simulink model "LFCSsimulink"  (R2015b)
settings: Solver=VariableStepAuto  StartTime=0.0  StopTime=40  RelTol=1e-3
libraries: simulink x1
settings Model: PauseTimes=1  Creator=Vamshi  LastModifiedBy=Vamshi

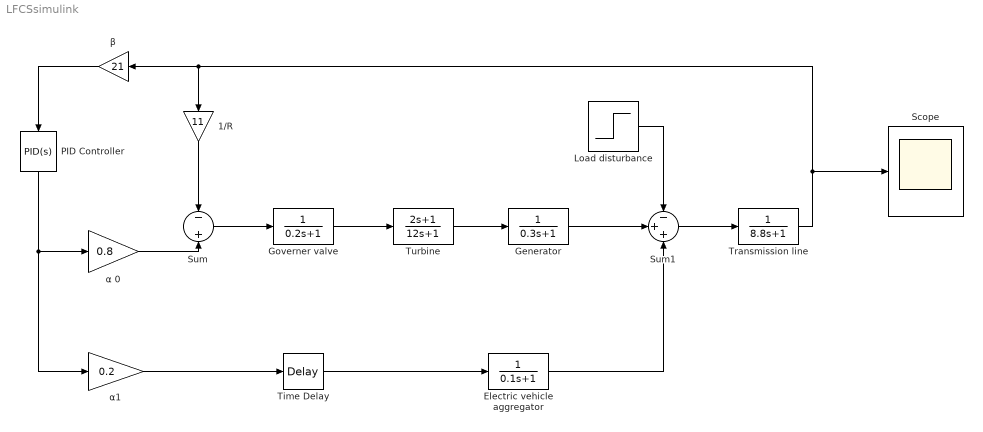
== system LFCSsimulink ==
  1/R : Gain  Gain=11
  Electric vehicle aggregator : TransferFcn  Denominator=[0.1 1]
  Generator : TransferFcn  Denominator=[0.3 1]
  Governer valve : TransferFcn  Denominator=[0.2 1]
  Load disturbance : Step  Time=0  After=.04  SampleTime=0
  PID Controller : simulink/Continuous/PID Controller  Controller=PID  TimeDomain=Continuous-time  SampleTime=-1  IntegratorMethod=Forward Euler  FilterMethod=Forward Euler  Form=Parallel  UseFilter=on  ControllerParametersSource=internal  P=-4  I=-2  D=0  N=100  InitialConditionSource=internal  InitialConditionForIntegrator=0  InitialConditionForFilter=0  ExternalReset=none  LimitOutput=off  UpperSaturationLimit=inf  LowerSaturationLimit=-inf  LinearizeAsGain=on  AntiWindupMode=none  Kb=1  TrackingMode=off  Kt=1  PParamMin=[]  PParamMax=[]  IParamMin=[]  IParamMax=[]  DParamMin=[]  DParamMax=[]  NParamMin=[]  NParamMax=[]  KbParamMin=[]  KbParamMax=[]  KtParamMin=[]  KtParamMax=[]  POutMin=[]  POutMax=[]  IOutMin=[]  IOutMax=[]  DOutMin=[]  DOutMax=[]  NOutMin=[]  NOutMax=[]  KbOutMin=[]  KbOutMax=[]  KtOutMin=[]  KtOutMax=[]  IntegratorOutMin=[]  IntegratorOutMax=[]  FilterOutMin=[]  FilterOutMax=[]  SumOutMin=[]  SumOutMax=[]  SumI1OutMin=[]  SumI1OutMax=[]  SumI2OutMin=[]  SumI2OutMax=[]  SumI3OutMin=[]  SumI3OutMax=[]  SumDOutMin=[]  SumDOutMax=[]  SaturationOutMin=[]  SaturationOutMax=[]  IntegratorContinuousStateAttributes=''  IntegratorStateMustResolveToSignalObject=off  IntegratorRTWStateStorageClass=Auto  FilterContinuousStateAttributes=''  FilterStateMustResolveToSignalObject=off  FilterRTWStateStorageClass=Auto  DifferentiatorICPrevScaledInput=0  DifferentiatorOutMin=[]  DifferentiatorOutMax=[]
  Scope : Scope
  Sum : Sum  Inputs=-+
  Sum1 : Sum  Inputs=-++
  Time Delay : TransportDelay  DelayTime=0.5  PadeOrder=5
  Transmission line : TransferFcn  Denominator=[8.8 1]
  Turbine : TransferFcn  Numerator=[2 1]  Denominator=[12 1]
  α 0 : Gain  Gain=0.8
  α1 : Gain  Gain=0.2
  β : Gain  Gain=21
  wires:
  Sum/1 -> Governer valve/1
  Governer valve/1 -> Turbine/1
  Turbine/1 -> Generator/1
  Generator/1 -> Sum1/2
  Sum1/1 -> Transmission line/1
  Load disturbance/1 -> Sum1/1
  α1/1 -> Time Delay/1
  1/R/1 -> Sum/1
  Transmission line/1 -> β/1, 1/R/1, Scope/1
  PID Controller/1 -> α1/1, α 0/1
  Electric vehicle aggregator/1 -> Sum1/3
  Time Delay/1 -> Electric vehicle aggregator/1
  β/1 -> PID Controller/1
  α 0/1 -> Sum/2
